simulink subsystem "Features_System"  (R2020b)
settings: Solver=VariableStepAuto  StartTime=0.0  StopTime=10.0  RelTol=1e-3
model mask{s0=[]}
settings Model: Creator=marco  LastModifiedBy=marco

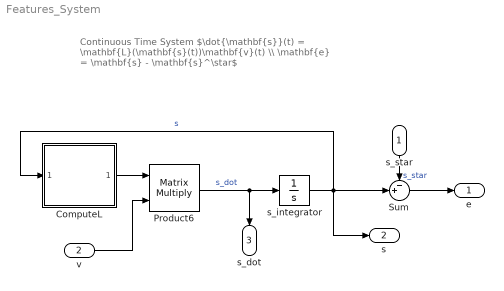
== system Features_System ==
  note: Continuous Time System
      | $\dot{\mathbf{s}}(t) = \mathbf{L}(\mathbf{s}(t))\mathbf{v}(t) \\ \mathbf{e} = \mathbf{s} - \mathbf{s}^\star$
  s_star : Inport
  v : Inport  Port=2
  ComputeL : Subsystem  ReferencedSubsystem=ComputeL
  Product6 : Product  Multiplication=Matrix(*)
  Sum : Sum  Inputs=-+|
  s_integrator : Integrator  InitialCondition=s0
  e : Outport
  s : Outport  Port=2
  s_dot : Outport  Port=3
  wires:
  Product6/1 -> s_dot/1, s_integrator/1  "s_dot"
  s_integrator/1 -> Sum/2, ComputeL/1, s/1  "s"
  s_star/1 -> Sum/1  "s_star"
  v/1 -> Product6/2
  Sum/1 -> e/1
  ComputeL/1 -> Product6/1
